simulink model "FICp"  (R2021b)
settings: Solver=VariableStepAuto  StartTime=0.0  StopTime=10.0  RelTol=1e-3
libraries: simulink_extras x1
settings Model: Creator=rapha  LastModifiedBy=Bianca
settings DataIOCC: ExternalInput=[clk, a, abs, jmp,b]  LoadExternalInput=on
settings HardwareCC: ProdBitPerPointer=32  ProdBitPerSizeT=32  ProdBitPerPtrDiffT=32  ProdWordSize=32  ProdLongLongMode=on  ProdHWDeviceType=RISC-V->RV32I
settings SFSimCC: SimCustomHeaderCode="#include \"header.h\""  SimUserSources=main.c
settings CodeAppCC: StateflowObjectComments=on

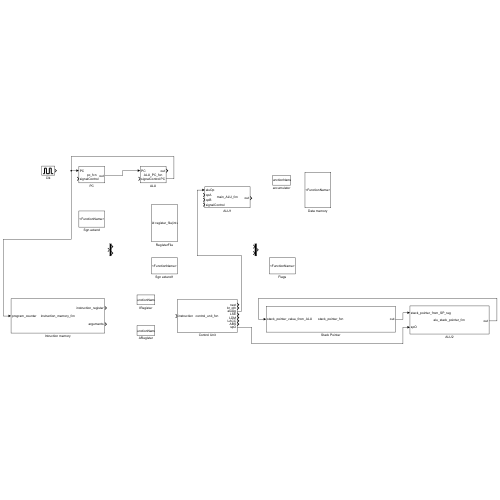
[thumbnail: Simulink's stored preview of the top-level diagram]
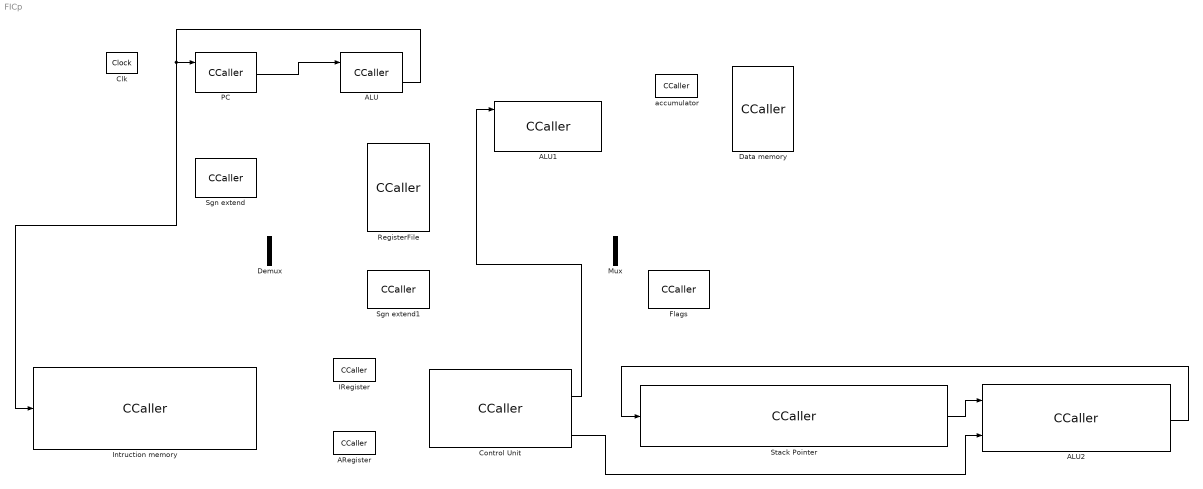
== system FICp ==
  ALU : CCaller  FunctionName=ALU_PC_fcn  PortSpecificationStruct="%)30     .    @ 4   8    (     @         %    \"     ,    !     0         %  0 \"0    $    _    07)G3F%M90  4&]R=$YA;64 4V-O<&4     26YD97@     5'EP90      4VEZ90      27-';&]B86P   X    P    !@    @    $          4    (     0    ,    !         !   P!O=70 #@   #     &    \"     0         !0    @    !     P    $         $  # &]U=  .    .     8    (    !          %    \"     $    &     0         0    !@   $]U='!U=   #@   #@    &    \"     8         !0    @    !     0    $         \"0    @               X    X    !@    @    $          4    (     0    8    !         !     &    =6EN=#$V   .    ,     8    (    !          %    \"     $    !     0         0  $ ,0    X    P    !@    @    ) @        4    (     0    $    !          (  0      #@   #     &    \"     0         !0    @    !     @    $         $  \" %!#   .    ,     8    (    !          %    \"     $    \"     0         0  ( 4$,   X   !     !@    @    $          4    (     0    L    !         !     +    26YP=71/=71P=70       X    X    !@    @    &          4    (     0    $    !          D    (               .    .     8    (    !          %    \"     $    %     0         0    !0   '5I;G0X    #@   #     &    \"     0         !0    @    !     @    $         $  \" \"TQ   .    ,     8    (    \"0(        %    \"     $    !     0         \"  $       X   !     !@    @    $          4    (     0    T    !         !     -    <VEG;F%L0V]N=')O;     X   !     !@    @    $          4    (     0    T    !         !     -    <VEG;F%L0V]N=')O;     X    X    !@    @    $          4    (     0    4    !         !     %    26YP=70    .    .     8    (    !@         %    \"     $    !     0         )    \"            / _#@   #@    &    \"     0         !0    @    !    !0    $         $     4   !U:6YT.     X    P    !@    @    $          4    (     0    $    !         !   0 Q    #@   #     &    \"     D\"        !0    @    !     0    $          @ !"
  ALU1 : CCaller  FunctionName=main_ALU_fcn  PortSpecificationStruct="%)30     .    T @   8    (     @         %    \"     4    !     0         %  0 \"0    $    _    07)G3F%M90  4&]R=$YA;64 4V-O<&4     26YD97@     5'EP90      4VEZ90      27-';&]B86P   X    P    !@    @    $          4    (     0    ,    !         !   P!O=70 #@   #     &    \"     0         !0    @    !     P    $         $  # &]U=  .    .     8    (    !          %    \"     $    &     0         0   ...(+2657 chars)"
  ALU2 : CCaller  FunctionName=alu_stack_pointer_fcn  PortSpecificationStruct="%)30     .    F 4   8    (     @         %    \"     ,    !     0         %  0 \"0    $    _    07)G3F%M90  4&]R=$YA;64 4V-O<&4     26YD97@     5'EP90      4VEZ90      27-';&]B86P   X    P    !@    @    $          4    (     0    ,    !         !   P!O=70 #@   #     &    \"     0         !0    @    !     P    $         $  # &]U=  .    .     8    (    !          %    \"     $    &     0         0    !@   $]U='!U=   #@   #@    &    \"     8         !0    @    !     0    $         \"0    @               X    X    !@    @    $          4    (     0    8    !         !     &    =6EN=#$V   .    ,     8    (    !          %    \"     $    !     0         0  $ ,0    X    P    !@    @    ) @        4    (     0    $    !          (  0      #@   %     &    \"     0         !0    @    !    &0    $         $    !D   !S=&%C:U]P;VEN=&5R7V9R;VU?4U!?<F5G          X   !0    !@    @    $          4    (     0   !D    !         !     9    <W1A8VM?<&]I;G1E<E]F<F]M7U-07W)E9P         .    .     8    (    !          %    \"     $    %     0         0    !0   $EN<'5T    #@   #@    &    \"     8         !0    @    !     0    $         \"0    @               X    X    !@    @    $          4    (     0    8    !         !     &    =6EN=#$V   .    ,     8    (    !          %    \"     $    !     0         0  $ ,0    X    P    !@    @    ) @        4    (     0    $    !          (  0      #@   #     &    \"     0         !0    @    !     P    $         $  # '-P3P .    ,     8    (    !          %    \"     $    #     0         0  , <W!/  X    X    !@    @    $          4    (     0    4    !         !     %    26YP=70    .    .     8    (    !@         %    \"     $    !     0         )    \"            / _#@   #@    &    \"     0         !0    @    !    !0    $         $     4   !U:6YT.     X    P    !@    @    $          4    (     0    $    !         !   0 Q    #@   #     &    \"     D\"        !0    @    !     0    $          @ !"
  ARegister : CCaller
  Clk : simulink_extras/Flip Flops/Clock  period=2
  Control Unit : CCaller  FunctionName=control_unit_fcn  PortSpecificationStruct="%)30     .    F \\   8    (     @         %    \"     D    !     0         %  0 \"0    $    _    07)G3F%M90  4&]R=$YA;64 4V-O<&4     26YD97@     5'EP90      4VEZ90      27-';&]B86P   X   !     !@    @    $          4    (     0    L    !         !     +    :6YS=')U8W1I;VX       X   !     !@    @    $          4    (     0    L    !         !     +    :6YS=')U8W1I;VX       X    X    !@    @    $    ...(+5001 chars)"
  Data memory : CCaller
  Demux : Demux  Outputs=2
  Flags : CCaller
  IRegister : CCaller
  Intruction memory : CCaller  FunctionName=instruction_memory_fcn  PortSpecificationStruct="%)30     .    V 4   8    (     @         %    \"     ,    !     0         %  0 \"0    $    _    07)G3F%M90  4&]R=$YA;64 4V-O<&4     26YD97@     5'EP90      4VEZ90      27-';&]B86P   X   !     !@    @    $          4    (     0    \\    !         !     /    <')O9W)A;5]C;W5N=&5R  X   !     !@    @    $          4    (     0    \\    !         !     /    <')O9W)A;5]C;W5N=&5R  X    X    !@    @    $   ...(+1632 chars)"
  Mux : Mux  Inputs=2
  PC : CCaller  FunctionName=pc_fcn  PortSpecificationStruct="%)30     .    > 4   8    (     @         %    \"     ,    !     0         %  0 \"0    $    _    07)G3F%M90  4&]R=$YA;64 4V-O<&4     26YD97@     5'EP90      4VEZ90      27-';&]B86P   X    P    !@    @    $          4    (     0    ,    !         !   P!O=70 #@   #     &    \"     0         !0    @    !     P    $         $  # &]U=  .    .     8    (    !          %    \"     $    &     0         0    !@   $]U='!U=   #@   #@    &    \"     8         !0    @    !     0    $         \"0    @               X    X    !@    @    $          4    (     0    8    !         !     &    =6EN=#$V   .    ,     8    (    !          %    \"     $    !     0         0  $ ,0    X    P    !@    @    ) @        4    (     0    $    !          (  0      #@   #     &    \"     0         !0    @    !     @    $         $  \" %!#   .    ,     8    (    !          %    \"     $    \"     0         0  ( 4$,   X    X    !@    @    $          4    (     0    4    !         !     %    26YP=70    .    .     8    (    !@         %    \"     $    !     0         )    \"               #@   #@    &    \"     0         !0    @    !    !0    $         $     4   !U:6YT.     X    P    !@    @    $          4    (     0    (    !         !   @ M,0  #@   #     &    \"     D\"        !0    @    !     0    $          @ !       .    0     8    (    !          %    \"     $    -     0         0    #0   '-I9VYA;$-O;G1R;VP    .    0     8    (    !          %    \"     $    -     0         0    #0   '-I9VYA;$-O;G1R;VP    .    .     8    (    !          %    \"     $    %     0         0    !0   $EN<'5T    #@   #@    &    \"     8         !0    @    !     0    $         \"0    @           #P/PX    X    !@    @    $          4    (     0    4    !         !     %    =6EN=#@    .    ,     8    (    !          %    \"     $    !     0         0  $ ,0    X    P    !@    @    ) @        4    (     0    $    !          (  0"
  RegisterFile : CCaller  FunctionName=void register_file(int a)
  Sgn extend : CCaller
  Sgn extend1 : CCaller
  Stack Pointer : CCaller  FunctionName=stack_pointer_fcn  PortSpecificationStruct="%)30     .    ^ ,   8    (     @         %    \"     (    !     0         %  0 \"0    $    _    07)G3F%M90  4&]R=$YA;64 4V-O<&4     26YD97@     5'EP90      4VEZ90      27-';&]B86P   X    P    !@    @    $          4    (     0    ,    !         !   P!O=70 #@   #     &    \"     0         !0    @    !     P    $         $  # &]U=  .    .     8    (    !          %    \"     $    &     0         0    !@   $]U='!U=   #@   #@    &    \"     8         !0    @    !     0    $         \"0    @               X    X    !@    @    $          4    (     0    8    !         !     &    =6EN=#$V   .    ,     8    (    !          %    \"     $    !     0         0  $ ,0    X    P    !@    @    ) @        4    (     0    $    !          (  0      #@   %     &    \"     0         !0    @    !    '     $         $    !P   !S=&%C:U]P;VEN=&5R7W9A;'5E7V9R;VU?04Q5      X   !0    !@    @    $          4    (     0   !P    !         !     <    <W1A8VM?<&]I;G1E<E]V86QU95]F<F]M7T%,50     .    .     8    (    !          %    \"     $    %     0         0    !0   $EN<'5T    #@   #@    &    \"     8         !0    @    !     0    $         \"0    @               X    X    !@    @    $          4    (     0    8    !         !     &    =6EN=#$V   .    ,     8    (    !          %    \"     $    !     0         0  $ ,0    X    P    !@    @    ) @        4    (     0    $    !          (  0"
  accumulator : CCaller
  wires:
  ALU2/1 -> Stack Pointer/1
  Stack Pointer/1 -> ALU2/1
  Control Unit/8 -> ALU2/2
  Control Unit/3 -> ALU1/1
  ALU/2 -> Intruction memory/1, PC/1
  PC/1 -> ALU/1
